simulink model "saccade"  (R2018b)
settings: Solver=VariableStepAuto  StartTime=0.0  StopTime=500  FixedStep=0.01  RelTol=1e-3  EnableMultiTasking=on
settings Model: Creator=huzy  LastModifiedBy=Jorish
settings OptimizationCC: LifeSpan=inf
settings DebuggingCC: SFUnexpectedBacktrackingDiag=warning  SFNoUnconditionalDefaultTransitionDiag=warning
settings SFSimCC: SimUseLocalCustomCode=off
settings RTWCC: RTWUseLocalCustomCode=off
settings CodeAppCC: StateflowObjectComments=on
settings GRTTargetCC: TargetLangStandard=C89/C90 (ANSI)  GeneratePreprocessorConditionals=Disable all
settings ConfigComp: CovMetricSettings=dw  CovHtmlReporting=on  CovSaveCumulativeToWorkspaceVar=on  CovSaveSingleToWorkspaceVar=on  CovExternalEMLEnable=off

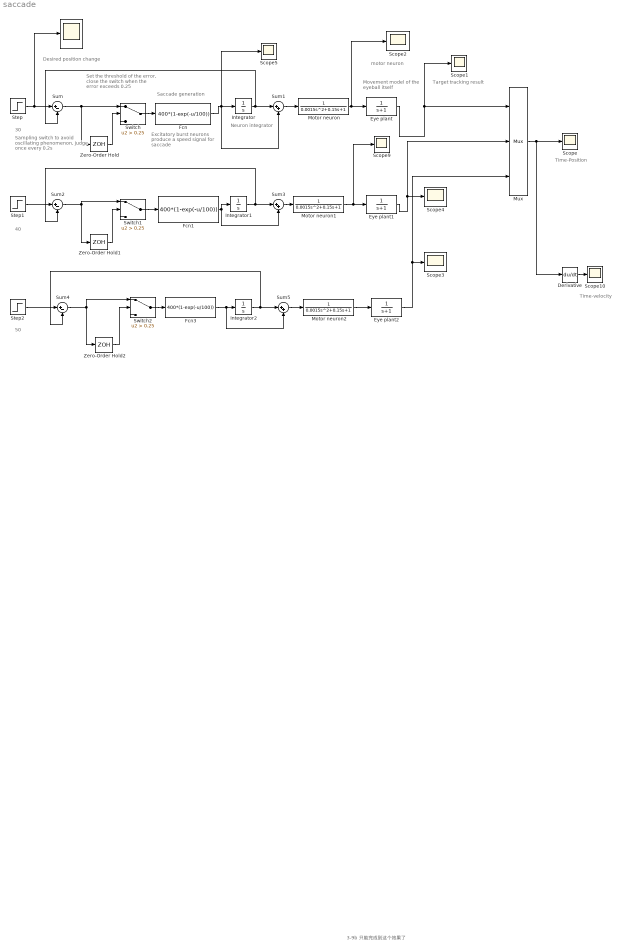
== system saccade ==
  note: motor neuron
  note: Sampling switch to avoid oscillating phenomenon, judge once every 0.2s
  note: Set the threshold of the error, close the switch when the error exceeds 0.25
  note: Excitatory burst neurons
      | produce a speed signal for saccade
  note: Movement model
      | of the eyeball itself
  note: 50
  note: 40
  note: 30
  note: 3-9b 只能完成到这个效果了
  note: Saccade generation
  note: Neuron
      | integrator
  note: Desired position change
  note: Target tracking result
  note: Time-Position
  note: Time-velocity
  " " : Scope
  Derivative : Derivative  CoefficientInTFapproximation=-1
  Eye plant : TransferFcn  Denominator=[1 1]
  Eye plant1 : TransferFcn  Denominator=[1 1]
  Eye plant2 : TransferFcn  Denominator=[1 1]
  Fcn : Fcn  Expr=400*(1-exp(-u/100))
  Fcn1 : Fcn  Expr=400*(1-exp(-u/100))
  Fcn3 : Fcn  Expr=400*(1-exp(-u/100))
  Integrator : Integrator
  Integrator1 : Integrator
  Integrator2 : Integrator
  Motor neuron : TransferFcn  Denominator=[0.0015 0.15 1]
  Motor neuron1 : TransferFcn  Denominator=[0.0015 0.15 1]
  Motor neuron2 : TransferFcn  Denominator=[0.0015 0.15 1]
  Mux : Mux  Inputs=3
  Scope{,1..5,9..10} (8 alike) : Scope
  Step : Step  Time=100  After=30  SampleTime=0
  Step1 : Step  Time=100  After=40  SampleTime=0
  Step2 : Step  Time=100  After=50  SampleTime=0
  Sum : Sum  Inputs=|+-
  Sum1 : Sum  Inputs=|++
  Sum2 : Sum  Inputs=|+-
  Sum3 : Sum  Inputs=|++
  Sum4 : Sum  Inputs=|+-
  Sum5 : Sum  Inputs=|++
  Switch : Switch  Criteria=u2 > Threshold  Threshold=0.25
  Switch1 : Switch  Criteria=u2 > Threshold  Threshold=0.25
  Switch2 : Switch  Criteria=u2 > Threshold  Threshold=0.25
  Zero-Order Hold : ZeroOrderHold  SampleTime=0.2
  Zero-Order Hold1 : ZeroOrderHold  SampleTime=0.2
  Zero-Order Hold2 : ZeroOrderHold  SampleTime=0.2
  wires:
  Integrator/1 -> Sum/2, Sum1/1
  Sum1/1 -> Motor neuron/1
  Eye plant/1 -> Mux/1, Scope1/1
  Sum/1 -> Switch/1, Zero-Order Hold/1
  Switch/1 -> Fcn/1
  Zero-Order Hold/1 -> Switch/2
  Fcn1/1 -> Integrator1/1, Sum3/2
  Integrator1/1 -> Sum2/2, Sum3/1
  Sum3/1 -> Motor neuron1/1
  Motor neuron1/1 -> Scope9/1, Eye plant1/1
  Step1/1 -> Sum2/1
  Sum2/1 -> Switch1/1, Zero-Order Hold1/1
  Switch1/1 -> Fcn1/1
  Zero-Order Hold1/1 -> Switch1/2
  Fcn3/1 -> Sum5/2, Integrator2/1
  Integrator2/1 -> Sum4/2, Sum5/1
  Sum5/1 -> Motor neuron2/1
  Motor neuron2/1 -> Eye plant2/1
  Step2/1 -> Sum4/1
  Sum4/1 -> Switch2/1, Zero-Order Hold2/1
  Switch2/1 -> Fcn3/1
  Zero-Order Hold2/1 -> Switch2/2
  Eye plant2/1 -> Mux/3, Scope3/1
  Eye plant1/1 -> Mux/2, Scope4/1
  Step/1 -> " "/1, Sum/1
  Fcn/1 -> Scope5/1, Sum1/2, Integrator/1
  Derivative/1 -> Scope10/1
  Motor neuron/1 -> Scope2/1, Eye plant/1
  Mux/1 -> Derivative/1, Scope/1
